simulink model "master_slave_lorenz_rossler2"  (R2018a)
settings: Solver=ode45  StartTime=0.0  StopTime=20  MaxStep=1e-2  RelTol=1e-3
libraries: simulink x1
settings Model: Creator=carma  LastModifiedBy=carma

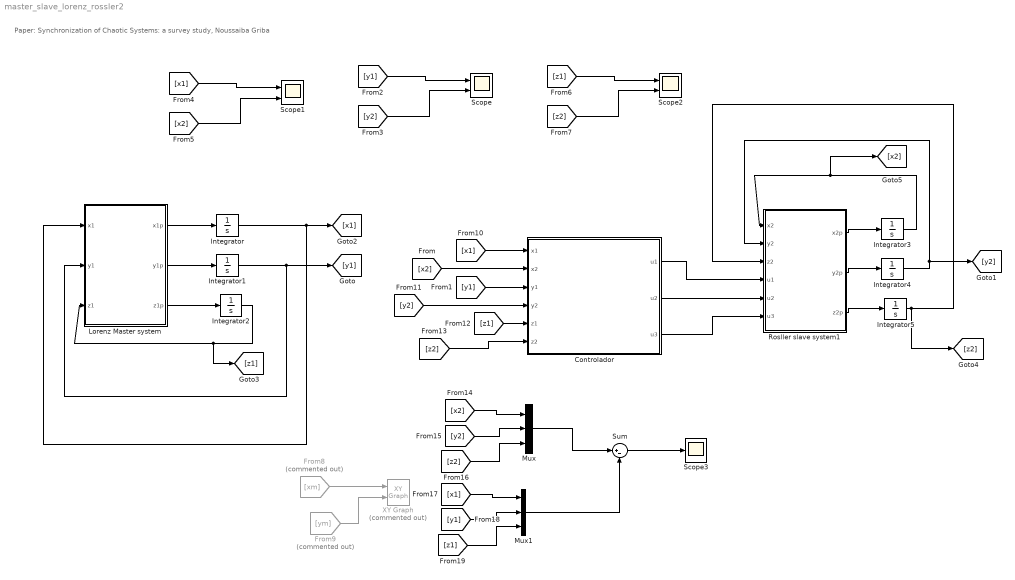
== system master_slave_lorenz_rossler2 ==
  note: Paper: Synchronization of Chaotic Systems: a survey study, Noussaiba Griba
  Controlador : MATLAB Function  TreatAsAtomicUnit=on
  From8 : From  Commented=on  GotoTag=xm
  From9 : From  Commented=on  GotoTag=ym
  Integrator : Integrator  InitialCondition=3
  Integrator1 : Integrator  InitialCondition=8
  Integrator2 : Integrator  InitialCondition=5
  Integrator3 : Integrator  InitialCondition=-3
  Integrator4 : Integrator  InitialCondition=-8
  Integrator5 : Integrator  InitialCondition=-5
  Lorenz Master system : MATLAB Function  TreatAsAtomicUnit=on
  Mux : Mux  Inputs=3
  Mux1 : Mux  Inputs=3
  Rosller slave system1 : MATLAB Function  TreatAsAtomicUnit=on
  Scope : Scope  NumInputPorts=2
  Scope1 : Scope  NumInputPorts=2
  Scope2 : Scope  NumInputPorts=2
  Scope3 : Scope
  Sum : Sum  Inputs=|+-
  XY Graph : simulink/Sinks/XY Graph  Commented=on  xmin=-5  xmax=6  ymin=-6  ymax=4  st=-1
  wires:
  Lorenz Master system/1(x1p) -> Integrator/1
  Lorenz Master system/2(y1p) -> Integrator1/1
  Lorenz Master system/3(z1p) -> Integrator2/1
  Integrator2/1 -> [z1], Lorenz Master system/3(z1)
  Integrator1/1 -> [y1], Lorenz Master system/2(y1)
  Rosller slave system1/2(y2p) -> Integrator4/1
  Rosller slave system1/3(z2p) -> Integrator5/1
  Rosller slave system1/1(x2p) -> Integrator3/1
  Integrator3/1 -> [x2], Rosller slave system1/1(x2)
  Integrator4/1 -> [y2], Rosller slave system1/2(y2)
  Integrator5/1 -> [z2], Rosller slave system1/3(z2)
  [x2] -> Controlador/2(x2)
  [y1] -> Controlador/3(y1)
  [y1] -> Scope/1
  [y2] -> Scope/2
  [x2] -> Scope1/2
  [x1] -> Scope1/1
  [z2] -> Scope2/2
  [z1] -> Scope2/1
  Integrator/1 -> [x1], Lorenz Master system/1(x1)
  From8/1 -> XY Graph/1
  From9/1 -> XY Graph/2
  [x1] -> Controlador/1(x1)
  [y2] -> Controlador/4(y2)
  [z1] -> Controlador/5(z1)
  [z2] -> Controlador/6(z2)
  Controlador/1(u1) -> Rosller slave system1/4(u1)
  Controlador/2(u2) -> Rosller slave system1/5(u2)
  Controlador/3(u3) -> Rosller slave system1/6(u3)
  [z1] -> Mux1/3
  Mux1/1 -> Sum/2
  [y1] -> Mux1/2
  [x1] -> Mux1/1
  [x2] -> Mux/1
  Mux/1 -> Sum/1
  [z2] -> Mux/3
  [y2] -> Mux/2
  Sum/1 -> Scope3/1

== matlab function master_slave_lorenz_rossler2/Rosller slave system1 ==
  data: x2 input; y2 input; z2 input; u1 input; x2p output; y2p output; z2p output; u2 input; u3 input
function [x2p,y2p,z2p] = fcn(x2,y2,z2,u1,u2,u3)

a=0.2;
b=0.2;
c=5.7;

x2p=-y2-z2+u1;
y2p=x2+a*y2+u2;
z2p=b+z2*(x2-c)+u3;

== matlab function master_slave_lorenz_rossler2/Lorenz Master system ==
  data: x1 input; x1p output; y1 input; z1 input; y1p output; z1p output
function [x1p,y1p,z1p] = fcn(x1,y1,z1)

s=10;
p=30;
b=8/3;


x1p=s*(y1-x1);
y1p=p*x1-y1-x1*z1;
z1p=x1*y1-b*z1

== matlab function master_slave_lorenz_rossler2/Controlador ==
  data: x1 input; u1 output; x2 input; y1 input; y2 input; z1 input; z2 input; u2 output; u3 output
function [u1,u2,u3] = fcn(x1,x2,y1,y2,z1,z2)

s=10;
p=30;
b=8/3;

a=0.2;
b2=0.2;
c=5.7;


ex=x2-x1;
ey=y2-y1;
ez=z2-z1;




u1=-s*x1+(s+1)*y1+z1-ex;
u2=-x1*z1+(p-1)*x1-(a+1)*y1-(a+1)*ey;
u3=ex*ez-x1*ez+x1*(y1-z1)-(ez+b-c)*z1-b2+ez;
